simulink model "hardwareTest"  (R2019a)
settings: Solver=FixedStepAuto  StartTime=0.0  StopTime=inf  RelTol=1e-3  EnableMultiTasking=on
libraries: simulink x2
settings Model: SimulationMode=external  Creator=florian  LastModifiedBy=florian
settings SolverCC: PositivePriorityOrder=on  AutoInsertRateTranBlk=on
settings OptimizationCC: EnhancedBackFolding=on  PassReuseOutputArgsAs=Individual arguments  MaxStackSize=64  OptimizeBlockOrder=speed  DifferentSizesBufferReuse=on  OptimizationCustomize=off
settings DebuggingCC: ParameterTunabilityLossMsg=error
settings HardwareCC: ProdBitPerPointer=32  ProdBitPerSizeT=32  ProdBitPerPtrDiffT=32  ProdLargestAtomicInteger=Long  ProdLargestAtomicFloat=Double  ProdWordSize=32  ProdLongLongMode=on  ProdHWDeviceType=ARM Compatible->ARM Cortex
settings SFSimCC: MATLABDynamicMemAlloc=off
settings RTWCC: SystemTargetFile=ert.tlc  HardwareBoard=Raspberry Pi  TLCOptions="-aInlineSetEventsForThisBaseRateFcn=TLC_FALSE -aSuppressMultiTaskScheduler=TLC_FALSE  -aRateBasedStepFcn=0"  TemplateMakefile=ert_default_tmf  GenerateReport=on  Toolchain=GNU GCC Raspberry Pi  BuildConfiguration=Faster Runs  IncludeHyperlinkInReport=on  LaunchReport=on  GenerateTraceInfo=on  GenerateTraceReport=on  GenerateTraceReportSl=on  GenerateTraceReportSf=on  GenerateTraceReportEml=on
settings CodeAppCC: ForceParamTrailComments=on  IgnoreCustomStorageClasses=off  OperatorAnnotations=on  SimulinkDataObjDesc=on  SFDataObjDesc=on  InsertBlockDesc=on
settings ERTTargetCC: SupportContinuousTime=on  SupportVariableSizeSignals=on  ExtMode=on  ExtModeTransport=2  ExtModeStaticAlloc=on  ExtModeMexFile=ext_xcp  ExtModeMexArgs='192.168.9.1' 0 17725  ExtModeIntrfLevel=Level2 - Open

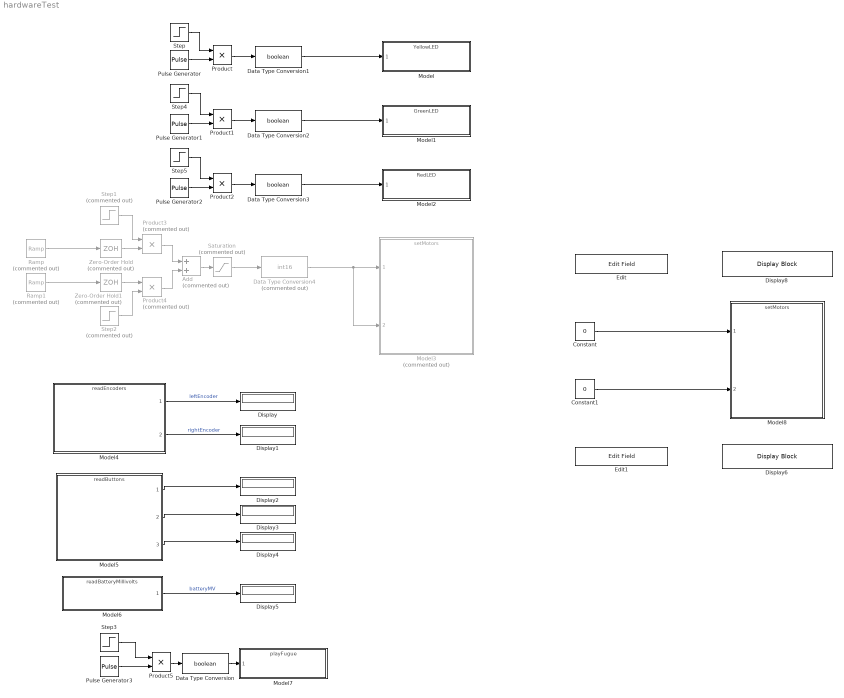
== system hardwareTest ==
  Add : Sum  Commented=on
  Constant : Constant  Value=0  OutMin=-1  OutMax=1  OutDataTypeStr=double
  Constant1 : Constant  Value=0  OutMin=-1  OutMax=1  OutDataTypeStr=double
  Data Type Conversion{,1..3} (4 alike) : DataTypeConversion  OutDataTypeStr=boolean
  Data Type Conversion4 : DataTypeConversion  Commented=on  OutDataTypeStr=int16
  Display{,1..5} (6 alike) : Display
  Display6 : DisplayBlock  LabelPosition=Hide  Format=short
  Display8 : DisplayBlock  LabelPosition=Hide  Format=short
  Edit : EditField  LabelPosition=Hide  ShowInitialText=on  Alignment=Center
  Edit1 : EditField  LabelPosition=Hide  ShowInitialText=on  Alignment=Center
  Model : ModelReference  ModelNameDialog=YellowLED.slx  SimulationMode=Normal  ModelReferenceVersion=1.18
  Model1 : ModelReference  ModelNameDialog=GreenLED.slx  SimulationMode=Normal  ModelReferenceVersion=1.9
  Model2 : ModelReference  ModelNameDialog=RedLED.slx  SimulationMode=Normal  ModelReferenceVersion=1.8
  Model3 : ModelReference  Commented=on  ModelNameDialog=setMotors.slx  SimulationMode=Normal  ModelReferenceVersion=1.5
  Model4 : ModelReference  ModelNameDialog=readEncoders.slx  SimulationMode=Normal  ModelReferenceVersion=1.5
  Model5 : ModelReference  ModelNameDialog=readButtons.slx  SimulationMode=Normal  ModelReferenceVersion=1.11
  Model6 : ModelReference  ModelNameDialog=readBatteryMillivolts  SimulationMode=Normal  ModelReferenceVersion=1.6
  Model7 : ModelReference  ModelNameDialog=playFugue.slx  SimulationMode=Normal  ModelReferenceVersion=1.10
  Model8 : ModelReference  ModelNameDialog=setMotors.slx  SimulationMode=Normal  ModelReferenceVersion=1.5
  Product{,1..2,5} (4 alike) : Product
  Product3 : Product  Commented=on
  Product4 : Product  Commented=on
  Pulse Generator : DiscretePulseGenerator  SampleTime=0.5
  Pulse Generator1 : DiscretePulseGenerator  SampleTime=0.1
  Pulse Generator2 : DiscretePulseGenerator  SampleTime=0.05
  Pulse Generator3 : DiscretePulseGenerator  Period=100  SampleTime=0.05
  Ramp : simulink/Sources/Ramp  Commented=on  slope=20  start=0  InitialOutput=0
  Ramp1 : simulink/Sources/Ramp  Commented=on  slope=-20  start=30  InitialOutput=0
  Saturation : Saturate  Commented=on  UpperLimit=400  LowerLimit=-400
  Step : Step  Time=15  Before=1  After=0  SampleTime=.5
  Step1 : Step  Commented=on  Time=25  Before=1  After=0  SampleTime=.1
  Step2 : Step  Commented=on  Time=55  Before=1  After=0  SampleTime=.1
  Step3 : Step  Time=0  Before=1  After=0  SampleTime=.05
  Step4 : Step  Time=15  Before=1  After=0  SampleTime=.1
  Step5 : Step  Time=15  Before=1  After=0  SampleTime=.05
  Zero-Order Hold : ZeroOrderHold  Commented=on  SampleTime=.1
  Zero-Order Hold1 : ZeroOrderHold  Commented=on  SampleTime=.1
  wires:
  Data Type Conversion1/1 -> Model/1
  Data Type Conversion2/1 -> Model1/1
  Data Type Conversion3/1 -> Model2/1
  Product/1 -> Data Type Conversion1/1
  Pulse Generator/1 -> Product/2
  Pulse Generator1/1 -> Product1/2
  Product1/1 -> Data Type Conversion2/1
  Step/1 -> Product/1
  Pulse Generator2/1 -> Product2/2
  Product2/1 -> Data Type Conversion3/1
  Saturation/1 -> Data Type Conversion4/1
  Step4/1 -> Product1/1
  Step5/1 -> Product2/1
  Ramp/1 -> Zero-Order Hold/1
  Ramp1/1 -> Zero-Order Hold1/1
  Step1/1 -> Product3/1
  Zero-Order Hold/1 -> Product3/2
  Add/1 -> Saturation/1
  Product3/1 -> Add/1
  Zero-Order Hold1/1 -> Product4/1
  Product4/1 -> Add/2
  Step2/1 -> Product4/2
  Model4/1 -> Display/1  "leftEncoder"
  Model4/2 -> Display1/1  "rightEncoder"
  Model6/1 -> Display5/1  "batteryMV"
  Product5/1 -> Data Type Conversion/1
  Step3/1 -> Product5/1
  Pulse Generator3/1 -> Product5/2
  Data Type Conversion/1 -> Model7/1
  Data Type Conversion4/1 -> Model3/2, Model3/1
  Constant/1 -> Model8/1
  Constant1/1 -> Model8/2
  Model5/3 -> Display4/1
  Model5/2 -> Display3/1
  Model5/1 -> Display2/1
